simulink model "TorqueVectoring"  (R2024b)
settings: Solver=FixedStepAuto  StartTime=0.0  StopTime=10.0  RelTol=1e-3  EnableMultiTasking=on
undefined symbols (not defined in the file): FTyreVerticalStaticFL, FTyreVerticalStaticFR, FTyreVerticalStaticRL, FTyreVerticalStaticRR, IYawInertia, lTrackWidth, lWheelbase, MMotorMinAllowed, MNominal, rGearboxRatio, rTyreRadius, tTorqueVectoringErrorCorrection
libraries: simulink x18
settings Model: DataDictionary=Master_Dictionary.sldd  EnableAccessToBaseWorkspace=off  Creator=torni  LastModifiedBy=Will
settings OptimizationCC: DefaultParameterBehavior=Inlined  EnhancedBackFolding=on  PassReuseOutputArgsAs=Individual arguments  ZeroExternalMemoryAtStartup=off  ZeroInternalMemoryAtStartup=off  MaxStackSize=8192  OptimizeBlockOrder=speed  DifferentSizesBufferReuse=on  OptimizationCustomize=off  EfficientTunableParamExpr=on
settings DebuggingCC: ParameterTunabilityLossMsg=error
settings HardwareCC: ProdBitPerPointer=32  ProdBitPerSizeT=32  ProdBitPerPtrDiffT=32  ProdLargestAtomicInteger=Long  ProdLargestAtomicFloat=Double  ProdWordSize=32  ProdLongLongMode=on  ProdHWDeviceType=ARM Compatible->ARM Cortex-M
settings SFSimCC: MATLABDynamicMemAlloc=off
settings RTWCC: Description=Embedded Coder  SystemTargetFile=ert.tlc  HardwareBoard=STM32H7xx Based (Single-core)  TemplateMakefile=ert_default_tmf  Toolchain=GNU Tools for ARM Embedded Processors
settings CodeAppCC: ForceParamTrailComments=on  IgnoreCustomStorageClasses=off  OperatorAnnotations=on  SimulinkDataObjDesc=on  SFDataObjDesc=on  InsertBlockDesc=on
settings ERTTargetCC: TargetLangStandard=C99 (ISO)  CodeReplacementLibrary=ARM Cortex-M  ExtModeTransport=3  ExtModeStaticAlloc=on  ExtModeStaticAllocSize=2048  ExtModeMexFile=ext_xcp  ExtModeIntrfLevel=Level2 - Open

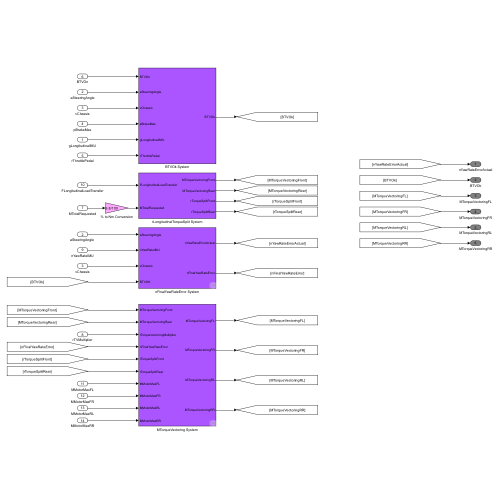
[thumbnail: Simulink's stored preview of the top-level diagram]
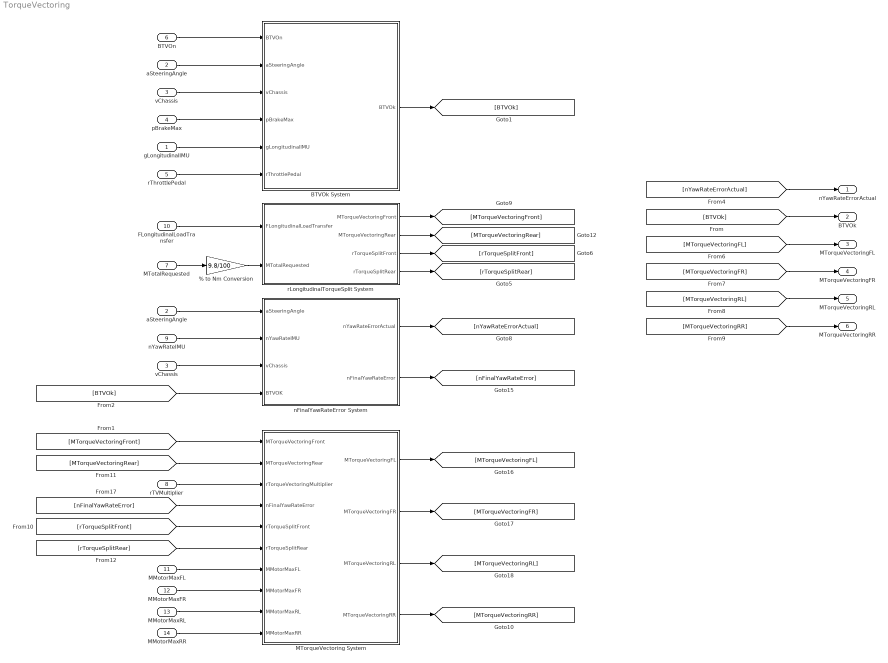
== system TorqueVectoring ==
  gLongitudinalIMU : Inport  OutDataTypeStr=double
  aSteeringAngle : Inport  Port=2  OutDataTypeStr=double
  vChassis : Inport  Port=3  OutDataTypeStr=double
  pBrakeMax : Inport  Port=4  OutDataTypeStr=double
  rThrottlePedal : Inport  Port=5  OutDataTypeStr=double
  BTVOn : Inport  Port=6  OutDataTypeStr=boolean
  MTotalRequested : Inport  Port=7  OutDataTypeStr=double
  rTVMultiplier : Inport  Port=8  OutDataTypeStr=double
  nYawRateIMU : Inport  Port=9  OutDataTypeStr=double
  FLongitudinalLoadTransfer : Inport  Port=10  OutDataTypeStr=double
  MMotorMaxFL : Inport  Port=11  OutDataTypeStr=double
  MMotorMaxFR : Inport  Port=12  OutDataTypeStr=double
  MMotorMaxRL : Inport  Port=13  OutDataTypeStr=double
  MMotorMaxRR : Inport  Port=14  OutDataTypeStr=double
  % to Nm Conversion : Gain  Gain=9.8/100
  BTVOk System : Subsystem
  MTorqueVectoring System : Subsystem
  "aSteeringAngle " : InportShadow  Port=2  OutDataTypeStr=double
  nFinalYawRateError System : Subsystem
  rLongitudinalTorqueSplit System : Subsystem
  "vChassis " : InportShadow  Port=3  OutDataTypeStr=double
  nYawRateErrorActual : Outport  OutDataTypeStr=double  VectorParamsAs1DForOutWhenUnconnected=off
  BTVOk : Outport  Port=2  OutDataTypeStr=boolean  VectorParamsAs1DForOutWhenUnconnected=off
  MTorqueVectoringFL : Outport  Port=3  OutDataTypeStr=double  VectorParamsAs1DForOutWhenUnconnected=off
  MTorqueVectoringFR : Outport  Port=4  OutDataTypeStr=double  VectorParamsAs1DForOutWhenUnconnected=off
  MTorqueVectoringRL : Outport  Port=5  OutDataTypeStr=double  VectorParamsAs1DForOutWhenUnconnected=off
  MTorqueVectoringRR : Outport  Port=6  OutDataTypeStr=double  VectorParamsAs1DForOutWhenUnconnected=off
  wires:
  MTorqueVectoring System/3(MTorqueVectoringRL) -> [MTorqueVectoringRL]
  % to Nm Conversion/1 -> rLongitudinalTorqueSplit System/2(MTotalRequested)
  [nFinalYawRateError] -> MTorqueVectoring System/4(nFinalYawRateError)
  MTotalRequested/1 -> % to Nm Conversion/1
  rLongitudinalTorqueSplit System/1(MTorqueVectoringFront) -> [MTorqueVectoringFront]
  MTorqueVectoring System/2(MTorqueVectoringFR) -> [MTorqueVectoringFR]
  MTorqueVectoring System/1(MTorqueVectoringFL) -> [MTorqueVectoringFL]
  rTVMultiplier/1 -> MTorqueVectoring System/3(rTorqueVectoringMultiplier)
  FLongitudinalLoadTransfer/1 -> rLongitudinalTorqueSplit System/1(FLongitudinalLoadTransfer)
  "aSteeringAngle "/1 -> nFinalYawRateError System/1(aSteeringAngle)
  rThrottlePedal/1 -> BTVOk System/6(rThrottlePedal)
  [MTorqueVectoringFR] -> MTorqueVectoringFR/1
  [BTVOk] -> nFinalYawRateError System/4(BTVOK)
  [MTorqueVectoringRL] -> MTorqueVectoringRL/1
  nFinalYawRateError System/1(nYawRateErrorActual) -> [nYawRateErrorActual]
  "vChassis "/1 -> nFinalYawRateError System/3(vChassis)
  nFinalYawRateError System/2(nFinalYawRateError) -> [nFinalYawRateError]
  [MTorqueVectoringRR] -> MTorqueVectoringRR/1
  pBrakeMax/1 -> BTVOk System/4(pBrakeMax)
  [nYawRateErrorActual] -> nYawRateErrorActual/1
  [BTVOk] -> BTVOk/1
  rLongitudinalTorqueSplit System/2(MTorqueVectoringRear) -> [MTorqueVectoringRear]
  [MTorqueVectoringRear] -> MTorqueVectoring System/2(MTorqueVectoringRear)
  [MTorqueVectoringFront] -> MTorqueVectoring System/1(MTorqueVectoringFront)
  MTorqueVectoring System/4(MTorqueVectoringRR) -> [MTorqueVectoringRR]
  gLongitudinalIMU/1 -> BTVOk System/5(gLongitudinalIMU)
  BTVOk System/1(BTVOk) -> [BTVOk]
  vChassis/1 -> BTVOk System/3(vChassis)
  aSteeringAngle/1 -> BTVOk System/2(aSteeringAngle)
  [MTorqueVectoringFL] -> MTorqueVectoringFL/1
  BTVOn/1 -> BTVOk System/1(BTVOn)
  rLongitudinalTorqueSplit System/3(rTorqueSplitFront) -> [rTorqueSplitFront]
  rLongitudinalTorqueSplit System/4(rTorqueSplitRear) -> [rTorqueSplitRear]
  [rTorqueSplitFront] -> MTorqueVectoring System/5(rTorqueSplitFront)
  [rTorqueSplitRear] -> MTorqueVectoring System/6(rTorqueSplitRear)
  nYawRateIMU/1 -> nFinalYawRateError System/2(nYawRateIMU)
  MMotorMaxFL/1 -> MTorqueVectoring System/7(MMotorMaxFL)
  MMotorMaxRL/1 -> MTorqueVectoring System/9(MMotorMaxRL)
  MMotorMaxFR/1 -> MTorqueVectoring System/8(MMotorMaxFR)
  MMotorMaxRR/1 -> MTorqueVectoring System/10(MMotorMaxRR)

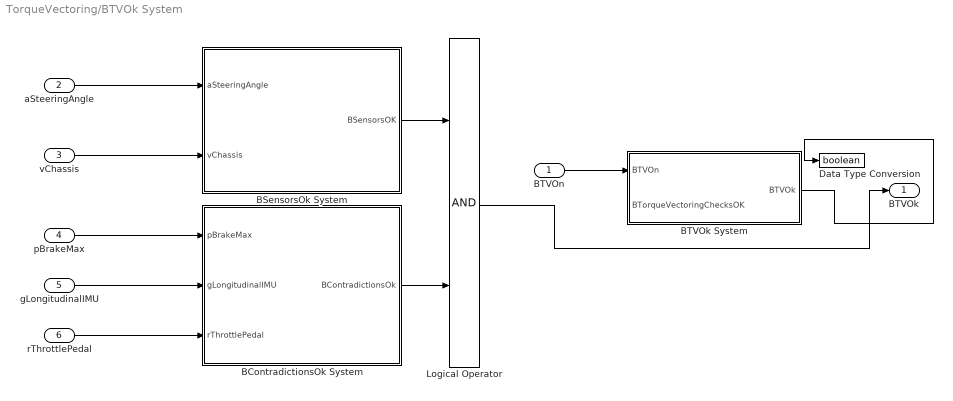
== system TorqueVectoring/BTVOk System ==
  BTVOn : Inport  OutDataTypeStr=boolean
  aSteeringAngle : Inport  Port=2  OutDataTypeStr=double
  vChassis : Inport  Port=3  OutDataTypeStr=double
  pBrakeMax : Inport  Port=4  OutDataTypeStr=double
  gLongitudinalIMU : Inport  Port=5  OutDataTypeStr=double
  rThrottlePedal : Inport  Port=6  OutDataTypeStr=double
  BContradictionsOk System : Subsystem
  BSensorsOk System : Subsystem
  BTVOk System : Stateflow chart  TreatAsAtomicUnit=on
  Data Type Conversion : DataTypeConversion  OutDataTypeStr=boolean  SaturateOnIntegerOverflow=off  RndMeth=Floor
  Logical Operator : Logic  AllPortsSameDT=off  OutDataTypeStr=boolean
  BTVOk : Outport  OutDataTypeStr=boolean  VectorParamsAs1DForOutWhenUnconnected=off
  wires:
  pBrakeMax/1 -> BContradictionsOk System/1(pBrakeMax)
  rThrottlePedal/1 -> BContradictionsOk System/3(rThrottlePedal)
  BTVOk System/1(BTVOk) -> Data Type Conversion/1
  BContradictionsOk System/1(BContradictionsOk) -> Logical Operator/2
  gLongitudinalIMU/1 -> BContradictionsOk System/2(gLongitudinalIMU)
  vChassis/1 -> BSensorsOk System/2(vChassis)
  BSensorsOk System/1(BSensorsOK) -> Logical Operator/1
  aSteeringAngle/1 -> BSensorsOk System/1(aSteeringAngle)
  BTVOn/1 -> BTVOk System/1(BTVOn)
  Logical Operator/1 -> BTVOk/1

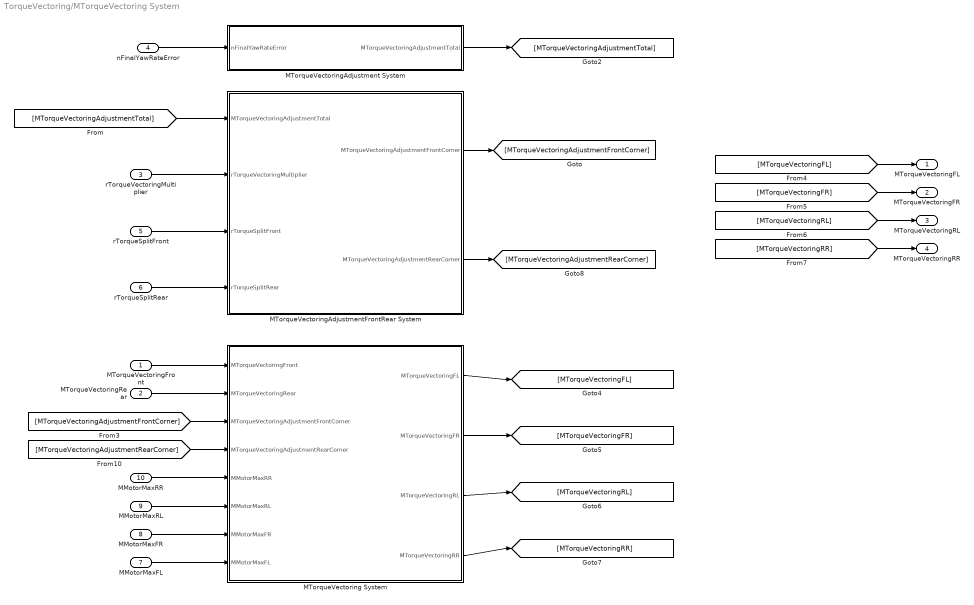
== system TorqueVectoring/MTorqueVectoring System ==
  MTorqueVectoringFront : Inport
  MTorqueVectoringRear : Inport  Port=2
  rTorqueVectoringMultiplier : Inport  Port=3  OutDataTypeStr=double
  nFinalYawRateError : Inport  Port=4  OutDataTypeStr=double
  rTorqueSplitFront : Inport  Port=5  OutDataTypeStr=double
  rTorqueSplitRear : Inport  Port=6  OutDataTypeStr=double
  MMotorMaxFL : Inport  Port=7  OutDataTypeStr=double
  MMotorMaxFR : Inport  Port=8  OutDataTypeStr=double
  MMotorMaxRL : Inport  Port=9  OutDataTypeStr=double
  MMotorMaxRR : Inport  Port=10  OutDataTypeStr=double
  MTorqueVectoring System : Subsystem
  MTorqueVectoringAdjustment System : Subsystem
  MTorqueVectoringAdjustmentFrontRear System : Subsystem
  MTorqueVectoringFL : Outport  OutDataTypeStr=double  VectorParamsAs1DForOutWhenUnconnected=off
  MTorqueVectoringFR : Outport  Port=2  OutDataTypeStr=double  VectorParamsAs1DForOutWhenUnconnected=off
  MTorqueVectoringRL : Outport  Port=3  OutDataTypeStr=double  VectorParamsAs1DForOutWhenUnconnected=off
  MTorqueVectoringRR : Outport  Port=4  OutDataTypeStr=double  VectorParamsAs1DForOutWhenUnconnected=off
  wires:
  [MTorqueVectoringAdjustmentRearCorner] -> MTorqueVectoring System/4("MTorqueVectoringAdjustmentRearCorner ")
  [MTorqueVectoringAdjustmentFrontCorner] -> MTorqueVectoring System/3(MTorqueVectoringAdjustmentFrontCorner)
  rTorqueSplitRear/1 -> MTorqueVectoringAdjustmentFrontRear System/4(rTorqueSplitRear)
  nFinalYawRateError/1 -> MTorqueVectoringAdjustment System/1(nFinalYawRateError)
  MTorqueVectoringAdjustment System/1(MTorqueVectoringAdjustmentTotal) -> [MTorqueVectoringAdjustmentTotal]
  [MTorqueVectoringAdjustmentTotal] -> MTorqueVectoringAdjustmentFrontRear System/1(MTorqueVectoringAdjustmentTotal)
  rTorqueVectoringMultiplier/1 -> MTorqueVectoringAdjustmentFrontRear System/2(rTorqueVectoringMultiplier)
  MTorqueVectoringFront/1 -> MTorqueVectoring System/1(MTorqueVectoringFront)
  MTorqueVectoringRear/1 -> MTorqueVectoring System/2(MTorqueVectoringRear)
  MTorqueVectoring System/1(MTorqueVectoringFL) -> [MTorqueVectoringFL]
  MTorqueVectoring System/2(MTorqueVectoringFR) -> [MTorqueVectoringFR]
  MTorqueVectoring System/3(MTorqueVectoringRL) -> [MTorqueVectoringRL]
  MTorqueVectoring System/4(MTorqueVectoringRR) -> [MTorqueVectoringRR]
  [MTorqueVectoringFL] -> MTorqueVectoringFL/1
  [MTorqueVectoringFR] -> MTorqueVectoringFR/1
  [MTorqueVectoringRL] -> MTorqueVectoringRL/1
  [MTorqueVectoringRR] -> MTorqueVectoringRR/1
  MTorqueVectoringAdjustmentFrontRear System/1(MTorqueVectoringAdjustmentFrontCorner) -> [MTorqueVectoringAdjustmentFrontCorner]
  MTorqueVectoringAdjustmentFrontRear System/2(MTorqueVectoringAdjustmentRearCorner) -> [MTorqueVectoringAdjustmentRearCorner]
  rTorqueSplitFront/1 -> MTorqueVectoringAdjustmentFrontRear System/3(rTorqueSplitFront)
  MMotorMaxFL/1 -> MTorqueVectoring System/8(MMotorMaxFL)
  MMotorMaxFR/1 -> MTorqueVectoring System/7(MMotorMaxFR)
  MMotorMaxRL/1 -> MTorqueVectoring System/6(MMotorMaxRL)
  MMotorMaxRR/1 -> MTorqueVectoring System/5(MMotorMaxRR)

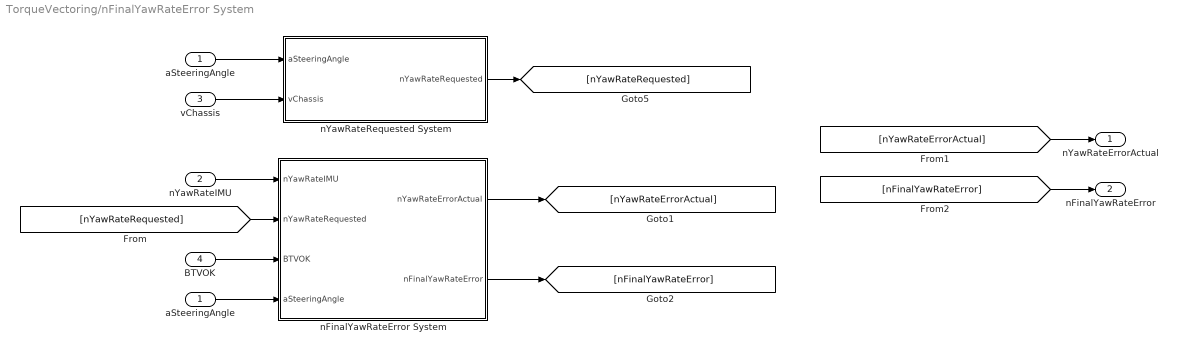
== system TorqueVectoring/nFinalYawRateError System ==
  aSteeringAngle : Inport  OutDataTypeStr=double
  nYawRateIMU : Inport  Port=2  OutDataTypeStr=double
  vChassis : Inport  Port=3  OutDataTypeStr=double
  BTVOK : Inport  Port=4  OutDataTypeStr=boolean
  "aSteeringAngle " : InportShadow  OutDataTypeStr=double
  nFinalYawRateError System : Subsystem
  nYawRateRequested System : Subsystem
  nYawRateErrorActual : Outport  OutDataTypeStr=double  VectorParamsAs1DForOutWhenUnconnected=off
  nFinalYawRateError : Outport  Port=2  OutDataTypeStr=double  VectorParamsAs1DForOutWhenUnconnected=off
  wires:
  nFinalYawRateError System/2(nFinalYawRateError) -> [nFinalYawRateError]
  aSteeringAngle/1 -> nYawRateRequested System/1(aSteeringAngle)
  vChassis/1 -> nYawRateRequested System/2(vChassis)
  nYawRateRequested System/1(nYawRateRequested) -> [nYawRateRequested]
  nYawRateIMU/1 -> nFinalYawRateError System/1(nYawRateIMU)
  [nYawRateRequested] -> nFinalYawRateError System/2(nYawRateRequested)
  BTVOK/1 -> nFinalYawRateError System/3(BTVOK)
  nFinalYawRateError System/1(nYawRateErrorActual) -> [nYawRateErrorActual]
  [nYawRateErrorActual] -> nYawRateErrorActual/1
  [nFinalYawRateError] -> nFinalYawRateError/1
  "aSteeringAngle "/1 -> nFinalYawRateError System/4("aSteeringAngle ")

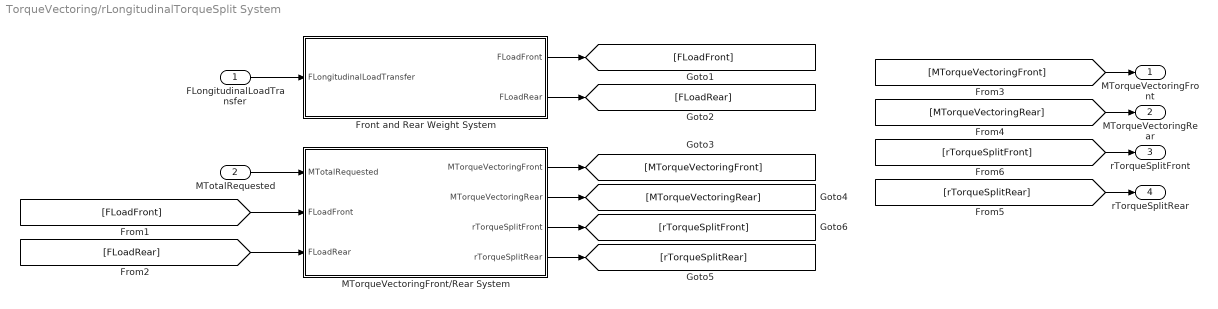
== system TorqueVectoring/rLongitudinalTorqueSplit System ==
  FLongitudinalLoadTransfer : Inport  OutDataTypeStr=double
  MTotalRequested : Inport  Port=2  OutDataTypeStr=double
  Front and Rear Weight System : Subsystem
  "MTorqueVectoringFront/Rear System " : Subsystem
  MTorqueVectoringFront : Outport  OutDataTypeStr=double  VectorParamsAs1DForOutWhenUnconnected=off
  MTorqueVectoringRear : Outport  Port=2  OutDataTypeStr=double  VectorParamsAs1DForOutWhenUnconnected=off
  rTorqueSplitFront : Outport  Port=3  OutDataTypeStr=double  VectorParamsAs1DForOutWhenUnconnected=off
  rTorqueSplitRear : Outport  Port=4  OutDataTypeStr=double  VectorParamsAs1DForOutWhenUnconnected=off
  wires:
  FLongitudinalLoadTransfer/1 -> Front and Rear Weight System/1(FLongitudinalLoadTransfer)
  Front and Rear Weight System/1(FLoadFront) -> [FLoadFront]
  Front and Rear Weight System/2(FLoadRear) -> [FLoadRear]
  MTotalRequested/1 -> "MTorqueVectoringFront/Rear System "/1(MTotalRequested)
  [FLoadFront] -> "MTorqueVectoringFront/Rear System "/2(FLoadFront)
  [FLoadRear] -> "MTorqueVectoringFront/Rear System "/3(FLoadRear)
  "MTorqueVectoringFront/Rear System "/1(MTorqueVectoringFront) -> [MTorqueVectoringFront]
  "MTorqueVectoringFront/Rear System "/2(MTorqueVectoringRear) -> [MTorqueVectoringRear]
  [MTorqueVectoringFront] -> MTorqueVectoringFront/1
  [MTorqueVectoringRear] -> MTorqueVectoringRear/1
  "MTorqueVectoringFront/Rear System "/3(rTorqueSplitFront) -> [rTorqueSplitFront]
  "MTorqueVectoringFront/Rear System "/4(rTorqueSplitRear) -> [rTorqueSplitRear]
  [rTorqueSplitFront] -> rTorqueSplitFront/1
  [rTorqueSplitRear] -> rTorqueSplitRear/1

== system TorqueVectoring/BTVOk System/BContradictionsOk System ==
  pBrakeMax : Inport  OutDataTypeStr=double
  gLongitudinalIMU : Inport  Port=2  OutDataTypeStr=double
  rThrottlePedal : Inport  Port=3  OutDataTypeStr=double
  BBrakeContradictionOk System : Subsystem
  BThrottleContradictionOk System : Subsystem
  Data Type Conversion : DataTypeConversion  OutDataTypeStr=boolean  SaturateOnIntegerOverflow=off  RndMeth=Floor
  Logical Operator : Logic  AllPortsSameDT=off  OutDataTypeStr=boolean
  BContradictionsOk : Outport  OutDataTypeStr=boolean  VectorParamsAs1DForOutWhenUnconnected=off
  wires:
  BThrottleContradictionOk System/1(BThrottleContradictionOk) -> Logical Operator/2
  BBrakeContradictionOk System/1(BBrakeContradictionOk) -> Logical Operator/1
  Logical Operator/1 -> Data Type Conversion/1
  pBrakeMax/1 -> BBrakeContradictionOk System/1(pBrakeMax)
  gLongitudinalIMU/1 -> BBrakeContradictionOk System/2(gLongitudinalIMU), BThrottleContradictionOk System/1(gLongitudinalIMU)
  rThrottlePedal/1 -> BThrottleContradictionOk System/2(rThrottlePedal)
  Data Type Conversion/1 -> BContradictionsOk/1

== system TorqueVectoring/BTVOk System/BSensorsOk System ==
  aSteeringAngle : Inport  OutDataTypeStr=double
  vChassis : Inport  Port=2  OutDataTypeStr=double
  BSteeringAngleOK System : Subsystem
  BVelocityOK System : Subsystem
  Logical Operator : Logic  AllPortsSameDT=off  OutDataTypeStr=boolean
  BSensorsOK : Outport  OutDataTypeStr=boolean  VectorParamsAs1DForOutWhenUnconnected=off
  wires:
  BVelocityOK System/1(BVelocityOK) -> Logical Operator/1
  BSteeringAngleOK System/1(BSteeringAngleOK) -> Logical Operator/2
  Logical Operator/1 -> BSensorsOK/1
  vChassis/1 -> BVelocityOK System/1(vChassis)
  aSteeringAngle/1 -> BSteeringAngleOK System/1(aSteeringAngle)

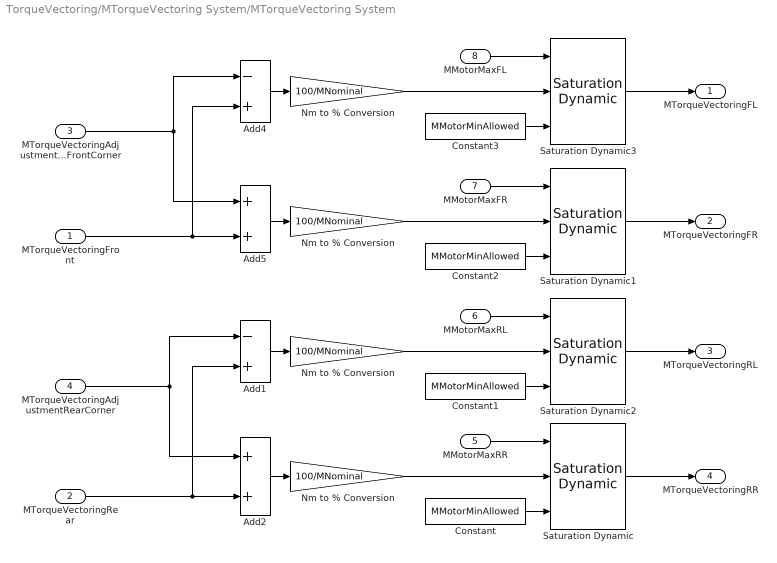
== system TorqueVectoring/MTorqueVectoring System/MTorqueVectoring System ==
  MTorqueVectoringFront : Inport  OutDataTypeStr=double
  MTorqueVectoringRear : Inport  Port=2  OutDataTypeStr=double
  MTorqueVectoringAdjustmentFrontCorner : Inport  Port=3  OutDataTypeStr=double
  "MTorqueVectoringAdjustmentRearCorner " : Inport  Port=4  OutDataTypeStr=double
  MMotorMaxRR : Inport  Port=5  OutDataTypeStr=double
  MMotorMaxRL : Inport  Port=6  OutDataTypeStr=double
  MMotorMaxFR : Inport  Port=7  OutDataTypeStr=double
  MMotorMaxFL : Inport  Port=8  OutDataTypeStr=double
  Add1 : Sum  Inputs=-+
  Add2 : Sum
  Add4 : Sum  Inputs=-+
  Add5 : Sum
  Constant{,1..3} (4 alike) : Constant  Value=MMotorMinAllowed
  Nm to % Conversion : Gain  Gain=100/MNominal
  "Nm to % Conversion " : Gain  Gain=100/MNominal
  "Nm to % Conversion " : Gain  Gain=100/MNominal
  "Nm to % Conversion " : Gain  Gain=100/MNominal
  Saturation Dynamic{,1..3} (4 alike) : simulink/Discontinuities/Saturation Dynamic  OutMin=[]  OutMax=[]  OutDataTypeStr=Inherit: Same as second input  OutDataType=fixdt(1, 16)  OutScaling=2^-10  DoSatur=off
  MTorqueVectoringFL : Outport  OutDataTypeStr=double  VectorParamsAs1DForOutWhenUnconnected=off
  MTorqueVectoringFR : Outport  Port=2  OutDataTypeStr=double  VectorParamsAs1DForOutWhenUnconnected=off
  MTorqueVectoringRL : Outport  Port=3  OutDataTypeStr=double  VectorParamsAs1DForOutWhenUnconnected=off
  MTorqueVectoringRR : Outport  Port=4  OutDataTypeStr=double  VectorParamsAs1DForOutWhenUnconnected=off
  wires:
  Add2/1 -> "Nm to % Conversion "/1
  Add4/1 -> Nm to % Conversion/1
  Add5/1 -> "Nm to % Conversion "/1
  Nm to % Conversion/1 -> Saturation Dynamic3/2
  MTorqueVectoringFront/1 -> Add4/2, Add5/2
  "Nm to % Conversion "/1 -> Saturation Dynamic/2
  MTorqueVectoringRear/1 -> Add1/2, Add2/2
  Saturation Dynamic2/1 -> MTorqueVectoringRL/1
  "Nm to % Conversion "/1 -> Saturation Dynamic2/2
  Saturation Dynamic/1 -> MTorqueVectoringRR/1
  Add1/1 -> "Nm to % Conversion "/1
  MTorqueVectoringAdjustmentFrontCorner/1 -> Add4/1, Add5/1
  "MTorqueVectoringAdjustmentRearCorner "/1 -> Add1/1, Add2/1
  Constant/1 -> Saturation Dynamic/3
  MMotorMaxRR/1 -> Saturation Dynamic/1
  MMotorMaxRL/1 -> Saturation Dynamic2/1
  Constant1/1 -> Saturation Dynamic2/3
  Constant2/1 -> Saturation Dynamic1/3
  MMotorMaxFR/1 -> Saturation Dynamic1/1
  "Nm to % Conversion "/1 -> Saturation Dynamic1/2
  Saturation Dynamic1/1 -> MTorqueVectoringFR/1
  Saturation Dynamic3/1 -> MTorqueVectoringFL/1
  Constant3/1 -> Saturation Dynamic3/3
  MMotorMaxFL/1 -> Saturation Dynamic3/1

== system TorqueVectoring/MTorqueVectoring System/MTorqueVectoringAdjustment System ==
  note: Torque (Nm) = (Yaw Rate Error (Rad/s) * Yaw Inertia (kgm2) * Tyre Radius(m)) / ( Gearbox Ratio * Time to Correct Error (s) 0.5*Track Width (m))
  nFinalYawRateError : Inport  OutDataTypeStr=double
  0.5 * Track width : Gain  Gain=1/(0.5*lTrackWidth)
  Saturation3 : Saturate  UpperLimit=80  LowerLimit=-80
  Time to correct error : Gain  Gain=1/tTorqueVectoringErrorCorrection
  Tyre Radius : Gain  Gain=rTyreRadius
  Tyre Radius1 : Gain  Gain=1/rGearboxRatio
  Yaw Inertia : Gain  Gain=IYawInertia
  degs/s to rads/s conversion : Gain  Gain=pi/180
  MTorqueVectoringAdjustmentTotal : Outport  OutDataTypeStr=double  VectorParamsAs1DForOutWhenUnconnected=off
  wires:
  Time to correct error/1 -> Yaw Inertia/1
  0.5 * Track width/1 -> Tyre Radius1/1
  degs/s to rads/s conversion/1 -> Time to correct error/1
  Yaw Inertia/1 -> 0.5 * Track width/1
  Tyre Radius/1 -> Saturation3/1
  nFinalYawRateError/1 -> degs/s to rads/s conversion/1
  Saturation3/1 -> MTorqueVectoringAdjustmentTotal/1
  Tyre Radius1/1 -> Tyre Radius/1

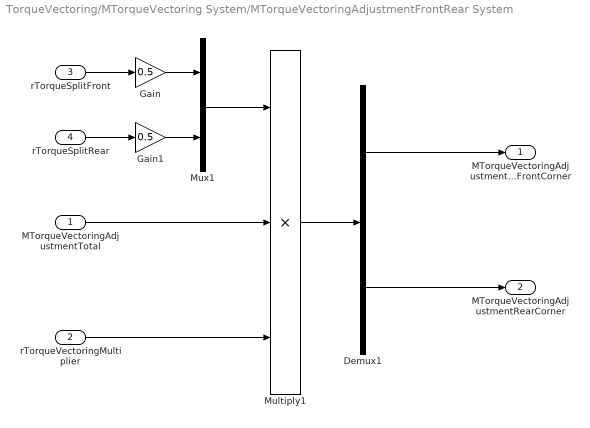
== system TorqueVectoring/MTorqueVectoring System/MTorqueVectoringAdjustmentFrontRear System ==
  MTorqueVectoringAdjustmentTotal : Inport  OutDataTypeStr=double
  rTorqueVectoringMultiplier : Inport  Port=2  OutDataTypeStr=double
  rTorqueSplitFront : Inport  Port=3  OutDataTypeStr=double
  rTorqueSplitRear : Inport  Port=4  OutDataTypeStr=double
  Demux1 : Demux  Outputs=2
  Gain : Gain  Gain=0.5
  Gain1 : Gain  Gain=0.5
  Multiply1 : Product  Inputs=3
  Mux1 : Mux  Inputs=2
  MTorqueVectoringAdjustmentFrontCorner : Outport  OutDataTypeStr=double  VectorParamsAs1DForOutWhenUnconnected=off
  MTorqueVectoringAdjustmentRearCorner : Outport  Port=2  OutDataTypeStr=double  VectorParamsAs1DForOutWhenUnconnected=off
  wires:
  Gain1/1 -> Mux1/2
  Gain/1 -> Mux1/1
  Demux1/1 -> MTorqueVectoringAdjustmentFrontCorner/1
  rTorqueSplitRear/1 -> Gain1/1
  Multiply1/1 -> Demux1/1
  Mux1/1 -> Multiply1/1
  MTorqueVectoringAdjustmentTotal/1 -> Multiply1/2
  rTorqueVectoringMultiplier/1 -> Multiply1/3
  Demux1/2 -> MTorqueVectoringAdjustmentRearCorner/1
  rTorqueSplitFront/1 -> Gain/1

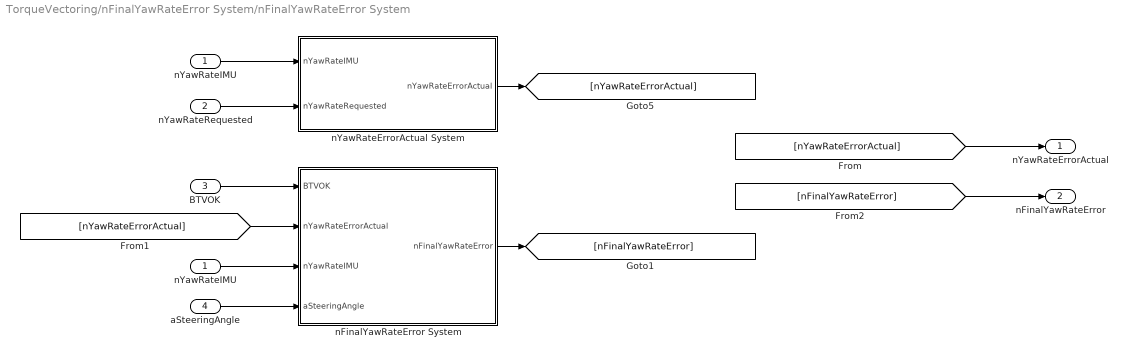
== system TorqueVectoring/nFinalYawRateError System/nFinalYawRateError System ==
  nYawRateIMU : Inport  OutDataTypeStr=double
  nYawRateRequested : Inport  Port=2  OutDataTypeStr=double
  BTVOK : Inport  Port=3  OutDataTypeStr=boolean
  "aSteeringAngle " : Inport  Port=4  OutDataTypeStr=double
  nFinalYawRateError System : Subsystem
  nYawRateErrorActual System : Subsystem
  "nYawRateIMU " : InportShadow  OutDataTypeStr=double
  nYawRateErrorActual : Outport  OutDataTypeStr=double  VectorParamsAs1DForOutWhenUnconnected=off
  nFinalYawRateError : Outport  Port=2  OutDataTypeStr=double  VectorParamsAs1DForOutWhenUnconnected=off
  wires:
  nYawRateErrorActual System/1(nYawRateErrorActual) -> [nYawRateErrorActual]
  nYawRateIMU/1 -> nYawRateErrorActual System/1(nYawRateIMU)
  nYawRateRequested/1 -> nYawRateErrorActual System/2(nYawRateRequested)
  BTVOK/1 -> nFinalYawRateError System/1(BTVOK)
  [nYawRateErrorActual] -> nFinalYawRateError System/2(nYawRateErrorActual)
  [nYawRateErrorActual] -> nYawRateErrorActual/1
  nFinalYawRateError System/1(nFinalYawRateError) -> [nFinalYawRateError]
  [nFinalYawRateError] -> nFinalYawRateError/1
  "aSteeringAngle "/1 -> nFinalYawRateError System/4(aSteeringAngle)
  "nYawRateIMU "/1 -> nFinalYawRateError System/3(nYawRateIMU)

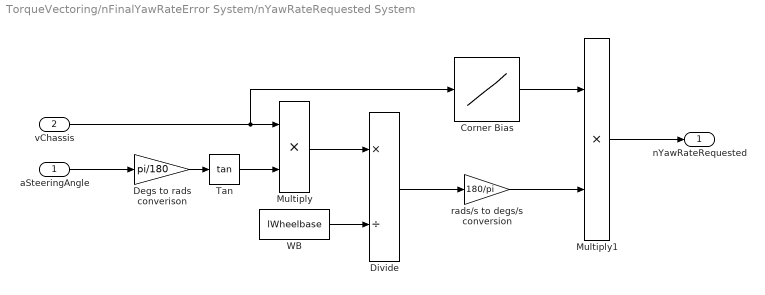
== system TorqueVectoring/nFinalYawRateError System/nYawRateRequested System ==
  aSteeringAngle : Inport  OutDataTypeStr=double
  vChassis : Inport  Port=2  OutDataTypeStr=double
  Corner Bias : Lookup_n-D  NumberOfTableDimensions=1  BreakpointsForDimension1=[0,5,10,15,20,25,30]  Table=[1.1,1.1,1.05,1,0.95,0.9,0.9]  InternalRulePriority=Speed  RndMeth=Simplest
  Degs to rads converison : Gain  Gain=pi/180
  Divide : Product  Inputs=*/  RndMeth=Zero  SaturateOnIntegerOverflow=on
  Multiply : Product
  Multiply1 : Product
  Tan : Trigonometry  Operator=tan
  WB : Constant  Value=lWheelbase
  rads/s to degs/s conversion : Gain  Gain=180/pi
  nYawRateRequested : Outport  OutDataTypeStr=double  VectorParamsAs1DForOutWhenUnconnected=off
  wires:
  WB/1 -> Divide/2
  Divide/1 -> rads/s to degs/s conversion/1
  Tan/1 -> Multiply/2
  vChassis/1 -> Corner Bias/1, Multiply/1
  Multiply/1 -> Divide/1
  Degs to rads converison/1 -> Tan/1
  aSteeringAngle/1 -> Degs to rads converison/1
  Corner Bias/1 -> Multiply1/1
  rads/s to degs/s conversion/1 -> Multiply1/2
  Multiply1/1 -> nYawRateRequested/1

== system TorqueVectoring/rLongitudinalTorqueSplit System/Front and Rear Weight System ==
  FLongitudinalLoadTransfer : Inport  OutDataTypeStr=double
  Add : Sum  Inputs=+-
  Add1 : Sum
  Add2 : Sum
  Add3 : Sum
  Constant : Constant  Value=FTyreVerticalStaticFL
  Constant1 : Constant  Value=FTyreVerticalStaticRL
  Constant2 : Constant  Value=FTyreVerticalStaticFR
  Constant3 : Constant  Value=FTyreVerticalStaticRR
  FLoadFront : Outport  OutDataTypeStr=double  VectorParamsAs1DForOutWhenUnconnected=off
  FLoadRear : Outport  Port=2  OutDataTypeStr=double  VectorParamsAs1DForOutWhenUnconnected=off
  wires:
  Add1/1 -> FLoadRear/1
  FLongitudinalLoadTransfer/1 -> Add1/1, Add/2
  Add/1 -> FLoadFront/1
  Add3/1 -> Add1/2
  Constant/1 -> Add2/1
  Constant2/1 -> Add2/2
  Add2/1 -> Add/1
  Constant1/1 -> Add3/1
  Constant3/1 -> Add3/2

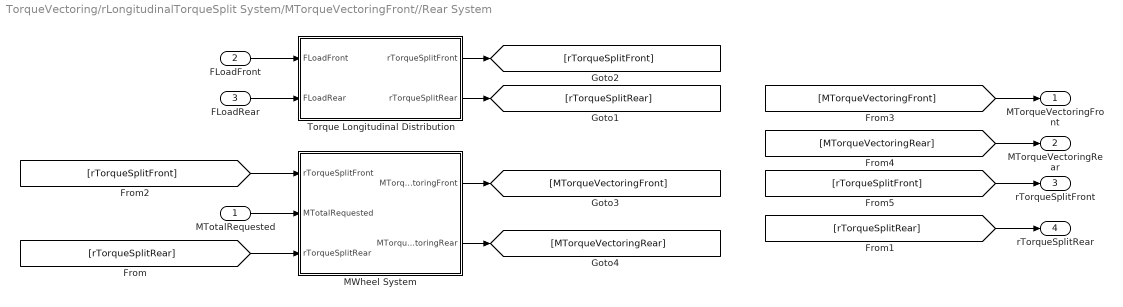
== system TorqueVectoring/rLongitudinalTorqueSplit System/MTorqueVectoringFront//Rear System  ==
  MTotalRequested : Inport  OutDataTypeStr=double
  FLoadFront : Inport  Port=2  OutDataTypeStr=double
  FLoadRear : Inport  Port=3  OutDataTypeStr=double
  MWheel System : Subsystem
  Torque Longitudinal Distribution : MATLAB Function  TreatAsAtomicUnit=on
  MTorqueVectoringFront : Outport  OutDataTypeStr=double  VectorParamsAs1DForOutWhenUnconnected=off
  MTorqueVectoringRear : Outport  Port=2  OutDataTypeStr=double  VectorParamsAs1DForOutWhenUnconnected=off
  rTorqueSplitFront : Outport  Port=3  OutDataTypeStr=double  VectorParamsAs1DForOutWhenUnconnected=off
  rTorqueSplitRear : Outport  Port=4  OutDataTypeStr=double  VectorParamsAs1DForOutWhenUnconnected=off
  wires:
  FLoadRear/1 -> Torque Longitudinal Distribution/2(FLoadRear)
  FLoadFront/1 -> Torque Longitudinal Distribution/1(FLoadFront)
  Torque Longitudinal Distribution/1(rTorqueSplitFront) -> [rTorqueSplitFront]
  Torque Longitudinal Distribution/2(rTorqueSplitRear) -> [rTorqueSplitRear]
  MTotalRequested/1 -> MWheel System/2(MTotalRequested)
  [rTorqueSplitFront] -> MWheel System/1(rTorqueSplitFront)
  [rTorqueSplitRear] -> MWheel System/3(rTorqueSplitRear)
  MWheel System/1(MTorqueVectoringFront) -> [MTorqueVectoringFront]
  [MTorqueVectoringFront] -> MTorqueVectoringFront/1
  MWheel System/2(MTorqueVectoringRear) -> [MTorqueVectoringRear]
  [MTorqueVectoringRear] -> MTorqueVectoringRear/1
  [rTorqueSplitRear] -> rTorqueSplitRear/1
  [rTorqueSplitFront] -> rTorqueSplitFront/1

== system TorqueVectoring/BTVOk System/BContradictionsOk System/BBrakeContradictionOk System ==
  pBrakeMax : Inport  OutDataTypeStr=double
  gLongitudinalIMU : Inport  Port=2  OutDataTypeStr=double
  Compare To Constant : simulink/Logic and Bit Operations/Compare To Constant  relop=>  const=10  OutDataTypeStr=boolean
  Compare To Constant1 : simulink/Logic and Bit Operations/Compare To Constant  relop=>  const=5  OutDataTypeStr=boolean
  Logical Operator1 : Logic  Operator=NAND  AllPortsSameDT=off  OutDataTypeStr=boolean
  BBrakeContradictionOk : Outport  OutDataTypeStr=boolean  VectorParamsAs1DForOutWhenUnconnected=off
  wires:
  Logical Operator1/1 -> BBrakeContradictionOk/1
  gLongitudinalIMU/1 -> Compare To Constant1/1
  Compare To Constant1/1 -> Logical Operator1/2
  Compare To Constant/1 -> Logical Operator1/1
  pBrakeMax/1 -> Compare To Constant/1

== system TorqueVectoring/BTVOk System/BContradictionsOk System/BThrottleContradictionOk System ==
  gLongitudinalIMU : Inport  OutDataTypeStr=double
  rThrottlePedal : Inport  Port=2  OutDataTypeStr=double
  Compare To Constant : simulink/Logic and Bit Operations/Compare To Constant  relop=>  const=80  OutDataTypeStr=boolean
  Compare To Constant1 : simulink/Logic and Bit Operations/Compare To Constant  relop=<  const=-5  OutDataTypeStr=boolean
  Logical Operator1 : Logic  Operator=NAND  AllPortsSameDT=off  OutDataTypeStr=boolean
  BThrottleContradictionOk : Outport  OutDataTypeStr=boolean  VectorParamsAs1DForOutWhenUnconnected=off
  wires:
  Logical Operator1/1 -> BThrottleContradictionOk/1
  rThrottlePedal/1 -> Compare To Constant/1
  Compare To Constant/1 -> Logical Operator1/1
  Compare To Constant1/1 -> Logical Operator1/2
  gLongitudinalIMU/1 -> Compare To Constant1/1

== system TorqueVectoring/BTVOk System/BSensorsOk System/BSteeringAngleOK System ==
  aSteeringAngle : Inport  OutDataTypeStr=double
  Compare To Constant : simulink/Logic and Bit Operations/Compare To Constant  relop=>  const=-29  OutDataTypeStr=boolean
  Compare To Constant1 : simulink/Logic and Bit Operations/Compare To Constant  relop=<  const=29  OutDataTypeStr=boolean
  Logical Operator : Logic  AllPortsSameDT=off  OutDataTypeStr=boolean
  BSteeringAngleOK : Outport  OutDataTypeStr=boolean  VectorParamsAs1DForOutWhenUnconnected=off
  wires:
  Logical Operator/1 -> BSteeringAngleOK/1
  aSteeringAngle/1 -> Compare To Constant/1, Compare To Constant1/1
  Compare To Constant/1 -> Logical Operator/1
  Compare To Constant1/1 -> Logical Operator/2

== system TorqueVectoring/BTVOk System/BSensorsOk System/BVelocityOK System ==
  vChassis : Inport  OutDataTypeStr=double
  Compare To Constant : simulink/Logic and Bit Operations/Compare To Constant  relop=>  const=-2  OutDataTypeStr=boolean
  Compare To Constant1 : simulink/Logic and Bit Operations/Compare To Constant  relop=<  const=31  OutDataTypeStr=boolean
  Logical Operator : Logic  AllPortsSameDT=off  OutDataTypeStr=boolean
  BVelocityOK : Outport  OutDataTypeStr=boolean  VectorParamsAs1DForOutWhenUnconnected=off
  wires:
  Compare To Constant/1 -> Logical Operator/2
  Compare To Constant1/1 -> Logical Operator/1
  Logical Operator/1 -> BVelocityOK/1
  vChassis/1 -> Compare To Constant1/1, Compare To Constant/1

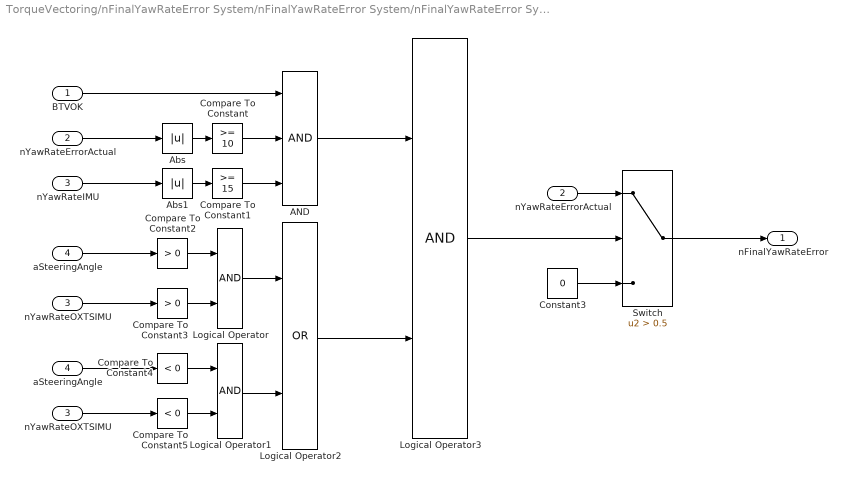
== system TorqueVectoring/nFinalYawRateError System/nFinalYawRateError System/nFinalYawRateError System ==
  BTVOK : Inport  OutDataTypeStr=boolean
  nYawRateErrorActual : Inport  Port=2  OutDataTypeStr=double
  nYawRateIMU : Inport  Port=3  OutDataTypeStr=double
  aSteeringAngle : Inport  Port=4  OutDataTypeStr=double
  AND : Logic  Inputs=3  AllPortsSameDT=off  OutDataTypeStr=boolean
  Abs : Abs  SaturateOnIntegerOverflow=off
  Abs1 : Abs  SaturateOnIntegerOverflow=off
  Compare To Constant : simulink/Logic and Bit Operations/Compare To Constant  relop=>=  const=10  OutDataTypeStr=boolean
  Compare To Constant1 : simulink/Logic and Bit Operations/Compare To Constant  relop=>=  const=15  OutDataTypeStr=boolean
  Compare To Constant2 : simulink/Logic and Bit Operations/Compare To Constant  relop=>  const=0  OutDataTypeStr=boolean
  Compare To Constant3 : simulink/Logic and Bit Operations/Compare To Constant  relop=>  const=0  OutDataTypeStr=boolean
  Compare To Constant4 : simulink/Logic and Bit Operations/Compare To Constant  relop=<  const=0  OutDataTypeStr=boolean
  Compare To Constant5 : simulink/Logic and Bit Operations/Compare To Constant  relop=<  const=0  OutDataTypeStr=boolean
  Constant3 : Constant  Value=0
  Logical Operator : Logic  AllPortsSameDT=off  OutDataTypeStr=boolean
  Logical Operator1 : Logic  AllPortsSameDT=off  OutDataTypeStr=boolean
  Logical Operator2 : Logic  Operator=OR  AllPortsSameDT=off  OutDataTypeStr=boolean
  Logical Operator3 : Logic  AllPortsSameDT=off  OutDataTypeStr=boolean
  Switch : Switch  Criteria=u2 > Threshold  Threshold=0.5  SaturateOnIntegerOverflow=off  InputSameDT=off
  "aSteeringAngle " : InportShadow  Port=4  OutDataTypeStr=double
  "nYawRateErrorActual " : InportShadow  Port=2  OutDataTypeStr=double
  "nYawRateOXTSIMU " : InportShadow  Port=3  OutDataTypeStr=double
  "nYawRateOXTSIMU " : InportShadow  Port=3  OutDataTypeStr=double
  nFinalYawRateError : Outport  OutDataTypeStr=double  VectorParamsAs1DForOutWhenUnconnected=off
  wires:
  Abs1/1 -> Compare To Constant1/1
  Compare To Constant1/1 -> AND/3
  Constant3/1 -> Switch/3
  Compare To Constant/1 -> AND/2
  Abs/1 -> Compare To Constant/1
  Switch/1 -> nFinalYawRateError/1
  Compare To Constant3/1 -> Logical Operator/2
  Logical Operator/1 -> Logical Operator2/1
  Compare To Constant4/1 -> Logical Operator1/1
  Compare To Constant5/1 -> Logical Operator1/2
  Compare To Constant2/1 -> Logical Operator/1
  Logical Operator1/1 -> Logical Operator2/2
  Logical Operator3/1 -> Switch/2
  AND/1 -> Logical Operator3/1
  Logical Operator2/1 -> Logical Operator3/2
  BTVOK/1 -> AND/1
  "nYawRateErrorActual "/1 -> Switch/1
  nYawRateErrorActual/1 -> Abs/1
  nYawRateIMU/1 -> Abs1/1
  aSteeringAngle/1 -> Compare To Constant2/1
  "nYawRateOXTSIMU "/1 -> Compare To Constant3/1
  "aSteeringAngle "/1 -> Compare To Constant4/1
  "nYawRateOXTSIMU "/1 -> Compare To Constant5/1

== system TorqueVectoring/nFinalYawRateError System/nFinalYawRateError System/nYawRateErrorActual System ==
  nYawRateIMU : Inport  OutDataTypeStr=double
  nYawRateRequested : Inport  Port=2  OutDataTypeStr=double
  Subtract : Sum  Inputs=-+
  nYawRateErrorActual : Outport  OutDataTypeStr=double  VectorParamsAs1DForOutWhenUnconnected=off
  wires:
  nYawRateIMU/1 -> Subtract/1
  nYawRateRequested/1 -> Subtract/2
  Subtract/1 -> nYawRateErrorActual/1

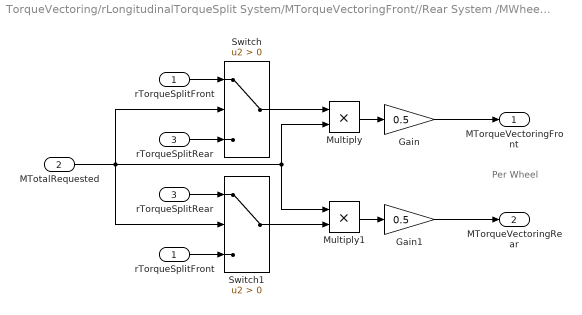
== system TorqueVectoring/rLongitudinalTorqueSplit System/MTorqueVectoringFront//Rear System /MWheel System ==
  note: Per Wheel
  rTorqueSplitFront : Inport  OutDataTypeStr=double
  MTotalRequested : Inport  Port=2  OutDataTypeStr=double
  rTorqueSplitRear : Inport  Port=3  OutDataTypeStr=double
  Gain : Gain  Gain=0.5
  Gain1 : Gain  Gain=0.5
  Multiply : Product
  Multiply1 : Product
  Switch : Switch  Criteria=u2 > Threshold  SaturateOnIntegerOverflow=off  InputSameDT=off
  Switch1 : Switch  Criteria=u2 > Threshold  SaturateOnIntegerOverflow=off  InputSameDT=off
  "rTorqueSplitFront " : InportShadow  OutDataTypeStr=double
  "rTorqueSplitRear " : InportShadow  Port=3  OutDataTypeStr=double
  MTorqueVectoringFront : Outport  OutDataTypeStr=double  VectorParamsAs1DForOutWhenUnconnected=off
  MTorqueVectoringRear : Outport  Port=2  OutDataTypeStr=double  VectorParamsAs1DForOutWhenUnconnected=off
  wires:
  Multiply1/1 -> Gain1/1
  Gain/1 -> MTorqueVectoringFront/1
  Gain1/1 -> MTorqueVectoringRear/1
  MTotalRequested/1 -> Multiply1/1, Multiply/2, Switch1/2, Switch/2
  Multiply/1 -> Gain/1
  rTorqueSplitFront/1 -> Switch/1
  Switch/1 -> Multiply/1
  rTorqueSplitRear/1 -> Switch/3
  Switch1/1 -> Multiply1/2
  "rTorqueSplitRear "/1 -> Switch1/1
  "rTorqueSplitFront "/1 -> Switch1/3

== stateflow chart TorqueVectoring/BTVOk System/BTVOk System ==
  state StartTV1
    BTVOk=1
  state StopTV
    BTVOk = 0
  StartTV1 -> StopTV : [BTorqueVectoringChecksOK<0.5]
  (default) -> StartTV1
  StopTV -> StartTV1 : [BTVOn<0.5]
  data: BTVOn input boolean; BTorqueVectoringChecksOK input boolean; BTVOk output double

== matlab function TorqueVectoring/rLongitudinalTorqueSplit System/MTorqueVectoringFront//Rear System /Torque Longitudinal Distribution ==
  data: FLoadFront input; rTorqueSplitFront output; FLoadRear input; rTorqueSplitRear output
function [rTorqueSplitFront,rTorqueSplitRear]= fcn(FLoadFront, FLoadRear)
rTorqueSplitFront = FLoadFront/(FLoadFront + FLoadRear);
rTorqueSplitRear = FLoadRear/(FLoadFront + FLoadRear);
